simulink library "lib_AirProps_ThermCond"  (R2015a)
settings: Solver=ode45  StartTime=0.0  StopTime=10.0  RelTol=1e-3
settings Model: Creator=jlkratz  LastModifiedBy=jlkratz

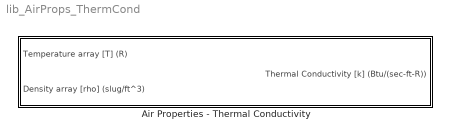
== system lib_AirProps_ThermCond ==
  Air Properties - Thermal Conductivity : Subsystem  mask(TSAT: Air Properties - Thermal Conductivity Block){BN_M=double(gcb)}
      mask prompts: BN_M "Block name"
      mask help:
      | This function provides an estimate of the thermal conductivity of air given its temperature and denisty. The function uses empirical relations which are valid for dry air in the temperature range of 60K - 2000K (108R - 3600R) and pressures up to 2000MPa. See the block help menu for details. This function is capable of evaluating the thermal conductivity for various temperature and density combinations at the same time given 1-D arrays of consistent lengths for both the temperature and density inputs.
      |
      | Units are clearly stated on the inport and outport so assure that your inputs are in the specified units and the output is properly converted to your desired units after the calculation.
      mask Help: web(which('AirProps_TSAT_ThermCond.html'),'-helpbrowser')

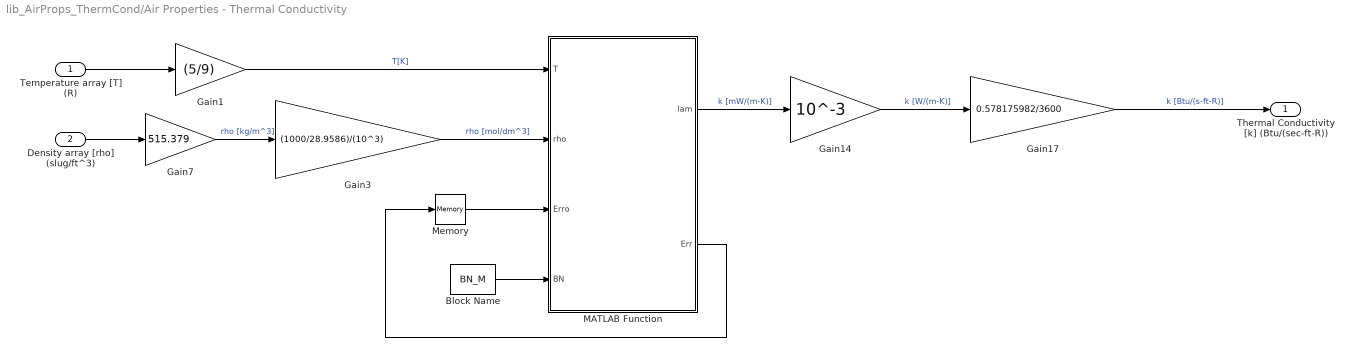
== system lib_AirProps_ThermCond/Air Properties - Thermal Conductivity ==
  Temperature array [T] (R) : Inport
  Density array [rho] (slug/ft^3) : Inport  Port=2
  Block Name : Constant  Value=BN_M
  Gain1 : Gain  Gain=(5/9)
  Gain14 : Gain  Gain=10^-3
  Gain17 : Gain  Gain=0.578175982/3600
  Gain3 : Gain  Gain=(1000/28.9586)/(10^3)
  Gain7 : Gain  Gain=515.379
  MATLAB Function : MATLAB Function  TreatAsAtomicUnit=on
  Memory : Memory  X0=zeros(1,3)
  Thermal Conductivity [k] (Btu/(sec-ft-R)) : Outport
  wires:
  Gain17/1 -> Thermal Conductivity [k] (Btu/(sec-ft-R))/1  "k [Btu/(s-ft-R)]"
  Gain14/1 -> Gain17/1  "k [W/(m-K)]"
  MATLAB Function/1(lam) -> Gain14/1  "k [mW/(m-K)]"
  Density array [rho] (slug/ft^3)/1 -> Gain7/1
  Gain7/1 -> Gain3/1  "rho [kg/m^3]"
  Gain3/1 -> MATLAB Function/2(rho)  "rho [mol/dm^3]"
  Block Name/1 -> MATLAB Function/4(BN)
  MATLAB Function/2(Err) -> Memory/1
  Memory/1 -> MATLAB Function/3(Erro)
  Gain1/1 -> MATLAB Function/1(T)  "T[K]"
  Temperature array [T] (R)/1 -> Gain1/1

== matlab function lib_AirProps_ThermCond/Air Properties - Thermal Conductivity/MATLAB Function ==
  data: T input; rho input; lam output; Erro input; BN input; Err output
function [lam,Err] = ThermCond_Air(T,rho,Erro,BN)
%#codegen

%Written By: Jonathan Kratz, NASA GRC
%Date: August 18, 2016
%Descirption: This function calculates the thermal conductivity of air 
%using empirical correlations from:
%   [1] Lemmon, E., Jacobsen, R., Penoncello, S., and Friend, D., 
%   Thermodynamic Properties of Air and Mixtures of Nitrogen, Argon, and 
%   Oxygen From 60 to 2000K at pressure to 2000MPa,” Journal of Physics 
%   Chemistry Reference Data, Vol. 29, No. 3, 2000.
%   [2] Lemmon, E., and Jacobsen, R., “Viscosity and Thermal Conductivity 
%   Equations for Nitrogen, Oxygen, Argon, and Air,” International Journal 
%   of Thermophysics, Vol. 25, No. 1, January 2004.
%
%Inputs:
%   T - Temperature array of the air in Kelvin (K)
%   rho - Density array of the air (mol/dm^3)
%
%Outputs:
%   k - Thermal conductivity array corresponding to T (mW/(m-K)) 

%Number of elements in set and array definitions
n = length(T);
m = length(rho);
Cp = zeros(1,n);
Cv = zeros(1,n);
mu0 = zeros(1,n);
mu = zeros(1,n);
drho_dp = zeros(1,n);
drho_dp_ref = zeros(1,n);
dalphar_ddel = zeros(1,n);
dalphar_ddel_ref = zeros(1,n);
d2alphar_ddel2 = zeros(1,n);
d2alphar_ddeldtau = zeros(1,n);
lam = zeros(1,n);

%error checking
Err = Erro;
ErrNum = 1;
if n ~= m && Erro(ErrNum) == 0
    Err(ErrNum) = 1;
    fprintf('warning in %s: The input arrays T and rho must be the same length.\n',char(BN));
end
if min(T) < 60 && Erro(ErrNum) == 0
    Err(ErrNum) = 1;
    fprintf('warning in %s: At least 1 element of the temperature array is below the temperature range (60-2000K, 108-3600R) which the empirical correlation is valid\n',char(BN));
end
ErrNum = ErrNum + 1;
if max(T) > 2000 && Erro(ErrNum) == 0
    Err(ErrNum) = 1;
    fprintf('warning in %s: At least 1 element of the temperature array is above the temperature range (60-2000K, 108-3600R) which the empirical correlation is valid\n',char(BN));
end

%parameters --------------------------------------------------------------%

Tc = 132.6312; %K
rhoc = 10.4477; %mol-dm^-3
R = 8.314510; %universal gas constant J/(mol-K)
M = 28.9586; %g/mol
pc = 3.78502; %MPa
Eo = 0.11; %nm
GAM = 0.055; %unitless
qD = 0.31; %nm
Tref = 2200; %K
PI = 3.14159; 
v = 0.63;
gamma = 1.2415;
R0 = 1.01;
ka = 1.380658*10^-23;
eps_k = 103.3; %K
sig = 0.360; %nm

%calculate viscosity -----------------------------------------------------%

for a = 1:n
    
    %Coefficients and exponents of the residual fluid viscosity equation
    N = [10.72, 1.122, 0.002019, -8.876, -0.02916];
    t = [0.2, 0.05, 2.4, 0.6, 3.6];
    d = [1, 4, 9, 1, 8];
    l = [0, 0, 0, 1, 1];

    %Coefficients of the Collision Integral Equation
    b = [0.431, -0.4623, 0.08406, 0.005341, -0.00331];

    for j = 1:n
        %Calculate dilute gas viscosity
        Tstar = T(a)/eps_k;
        CIEsum = 0;
        for i = 1:5
            CIEsum = CIEsum + b(i)*log(Tstar)^(i-1);
        end
        OMEGA = exp(CIEsum);
        mu0(a) = (0.0266958*(M*T(a))^0.5)/(sig^2*OMEGA);
        %Calculate the residual gas viscosity
        mur = 0;
        gam = 0;
        for i = 1:5
            if l(i) == 0
                gam = 0;
            else
                gam = 1;
            end
            mur = mur + N(i)*(Tc/T(a))^t(i)*(rho(a)/rhoc)^d(i)*exp(-gam*(rho(a)/rhoc)^l(i));
        end
        %Calculate the overall viscosity
        mu(a) = mu0(a) + mur; %10^-6 Pa-s
    end
    
end

%calculate Helmholtz deriviatives ----------------------------------------%

%Coefficients and exponents for the equation of state for air
N = [0.118160747229, 0.713116392079, -1.61824192067, 0.0714140178971, -0.0865421396646, 0.134211176704, 0.0112626704218, -0.0420533228842, 0.0349008431982, 0.000164957183186, -0.101365037921, -0.173813690970, -0.0472103183731, -0.0122523554253, -0.146629609713, -0.0316055879821, 0.000233594806142, 0.0148287891978, -0.00938782884667];
i = [1.0, 1.0, 1.0, 2.0, 3.0, 3.0, 4.0, 4.0, 4.0, 6.0, 1.0, 3.0, 5.0, 6.0, 1.0, 3.0, 11.0, 1.0, 3.0];
j = [0.0, 0.33, 1.01, 0.0, 0.0, 0.15, 0.0, 0.2, 0.35, 1.35, 1.6, 0.8, 0.95, 1.25, 3.6, 6.0, 3.25, 3.5, 15.0];
l = [0.0, 0.0, 0.0, 0.0, 0.0, 0.0, 0.0, 0.0, 0.0, 0.0, 1.0, 1.0, 1.0, 1.0, 2.0, 2.0, 2.0, 3.0, 3.0];

%First derivative of residual Helmholtz energy with respect to rho/rhoc
%for T
for a = 1:n
    sum1 = 0;
    for k = 1:10
        sum1 = sum1 + i(k)*N(k)*(rho(a)/rhoc)^(i(k)-1)*(Tc/T(a))^j(k);
    end
    sum2 = 0;
    for k = 11:19
        sum2 = sum2 + i(k)*N(k)*(rho(a)/rhoc)^(i(k)-1)*(Tc/T(a))^j(k)*exp((rho(a)/rhoc)^l(k))*(i(k)-l(k)*(rho(a)/rhoc)^l(k));
    end
    dalphar_ddel(a) = sum1 + sum2;
end
%for Tref
for a = 1:n
    sum1 = 0;
    for k = 1:10
        sum1 = sum1 + i(k)*N(k)*(rho(a)/rhoc)^(i(k)-1)*(Tc/Tref)^j(k);
    end
    sum2 = 0;
    for k = 11:19
        sum2 = sum2 + i(k)*N(k)*(rho(a)/rhoc)^(i(k)-1)*(Tc/Tref)^j(k)*exp((rho(a)/rhoc)^l(k))*(i(k)-l(k)*(rho(a)/rhoc)^l(k));
    end
    dalphar_ddel_ref(a) = sum1 + sum2;
end

%Second derivative of residual Helmholtz energy with respect to rho/rhoc
for a = 1:n
    sum1 = 0;
    for k = 1:10
        sum1 = sum1 + i(k)*(i(k)-1)*N(k)*(rho(a)/rhoc)^(i(k)-2)*(Tc/T(a))^j(k);
    end
    sum2 = 0;
    for k = 11:19
        sum2 = sum2 + N(k)*(rho(a)/rhoc)^(i(k)-2)*(Tc/T(a))^j(k)*exp(-(rho(a)/rhoc)^l(k))*((i(k)-l(k)*(rho(a)/rhoc)^l(k))*(i(k)-1-l(k)*(rho(a)/rhoc)^l(k))-l(k)^2*(rho(a)/rhoc)^l(k));
    end
    d2alphar_ddel2(a) = sum1 + sum2;
end

%Mixed derivative of residual Helmholtz energy
for a = 1:n
    sum1 = 0;
    for k = 1:10
        sum1 = sum1 + i(k)*j(k)*N(k)*(rho(a)/rhoc)^(i(k)-1)*(Tc/T(a))^(j(k)-1);
    end
    sum2 = 0;
    for k = 11:19
        sum2 = sum2 + j(k)*N(k)*(rho(a)/rhoc)^(i(k)-1)*(Tc/T(a))^(j(k)-1)*exp(-(rho(a)/rhoc)^l(k))*(i(k)-l(k)*(rho(a)/rhoc)^l(k));
    end
    d2alphar_ddeldtau(a) = sum1 + sum2;
end

%calculate heat capacity (Cp) --------------------------------------------%

%Coefficients of ideal gas expressions
N = [3.490888032, 2.395525583e-6, 7.172111248e-9, -3.115413101e-13, 0.223806688, 0.791309509, 0.212236768, 0.197938904, 3364.011, 2242.45, 11580.4];

for i = 1:n
    %Simplification variables
    u = N(9)/T(i);
    v = N(10)/T(i);
    w = N(11)/T(i);
    %Calculation of Cp (J/mol-K)
    sum = 0;
    for j = 1:4
        sum = sum + N(j)*T(i)^(j-1);
    end
    Cp(i) = R*(sum + N(5)/T(i)^1.5 + (N(6)*u^2.0*exp(u))/(exp(u)-1)^2.0 + (N(7)*v^2.0*exp(v))/((exp(v)-1)^2.0) + ((2.0/3.0)*N(8)*w^2.0*exp(-w))/((2.0/3.0)*exp(-w)+1)^2.0);
end

%calculate the heat capacity at constant volume (Cv) ---------------------%

%Cv (J/mol-K)
for i = 1:n
    Cv(i) = Cp(i) - R * ( (1 + (rho(i)/rhoc)*dalphar_ddel(i) - (rho(i)/rhoc)*(Tc/T(i))*d2alphar_ddeldtau(i))^2 / (1 + 2*(rho(i)/rhoc)*dalphar_ddel(i) + (rho(i)/rhoc)^2*d2alphar_ddel2(i)) );
end

%calculate drho/dp for T and Tref ----------------------------------------%

% for T
for a = 1:n
    drho_dp(a) = (1/(R*T(a)))*(1 + (rho(a)/rhoc)*dalphar_ddel(a))^-1;
end

% for Tref
for a = 1:n
    drho_dp_ref(a) = (1/(R*Tref))*(1 + (rho(a)/rhoc)*dalphar_ddel_ref(a))^-1;
end

%calculate thermal conductivity ------------------------------------------%

%Coefficients and exponents of the residual thermal conductivity equations
Nc = [1.308, 1.405, -1.036, 8.743, 14.76, -16.62, 3.793, -6.142, -0.3778];
tc = [0.0, -1.1, -0.3, 0.1, 0.0, 0.5, 2.7, 0.3, 1.3];
dc = [0, 0, 0, 1, 2, 3, 7, 7, 11];
lc = [0, 0, 0, 0, 0, 2, 2, 2, 2];

for a = 1:n
    %Dilute gas conductivity
    lam0 = Nc(1)*mu0(a) + Nc(2)*(Tc/T(a))^tc(2) + Nc(3)*(Tc/T(a))^tc(3);
    %Residual gas conductivity
    lamr = 0;
    gamc = 0;
    for i = 3:9
        if lc(i) == 0
            gamc = 0;
        else
            gamc = 1;
        end
        lamr = lamr +  Nc(i)*(Tc/T(a))^tc(i)*(rho(a)/rhoc)^dc(i)*exp(-gamc*(rho(a)/rhoc)^lc(i));
    end
    %Thermal conductivity critical enhancement model
    X = ((pc*rho(a))/rhoc^2)*drho_dp(a);
    XREF = ((pc*rho(a))/rhoc^2)*drho_dp_ref(a);
    E = Eo*((1/GAM)*(X-XREF*(Tref/T(a))))^(v/gamma);
    OMEGA_TIL = (2/PI)*(((Cp(a)-Cv(a))/Cp(a))*atan(E/qD) + (Cv(a)/Cp(a))*(E/qD));
    OMEGA0_TIL = (2/PI)*(1 - exp(-1/(qD/E + (1.0/3.0)*(E/qD)^2*(rhoc/rho(a))^2)));
    lamc = rho(a)*Cp(a)*((ka*R0*T(a))/(6*PI*E*mu(a)))*(OMEGA_TIL - OMEGA0_TIL);
    %Overall Thermal Conductivity
    lam(a) = lam0 + lamr + lamc; %mW/(m-K)
end
